simulink model "STATE_PROJECT"  (R2022b)
settings: Solver=FixedStepAuto  StartTime=0.0  StopTime=120.0  FixedStep=0.1  RelTol=1e-3
settings Model: Creator=alfon  LastModifiedBy=alfon

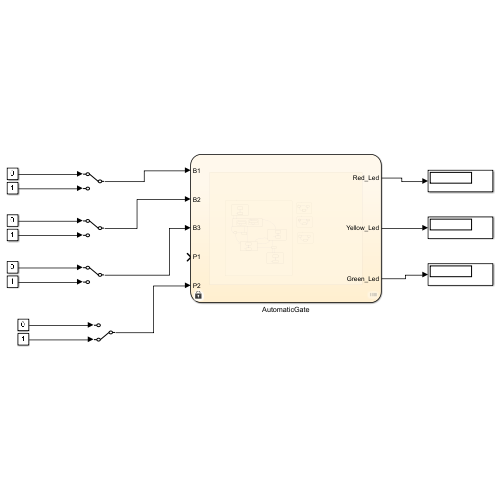
[thumbnail: Simulink's stored preview of the top-level diagram]
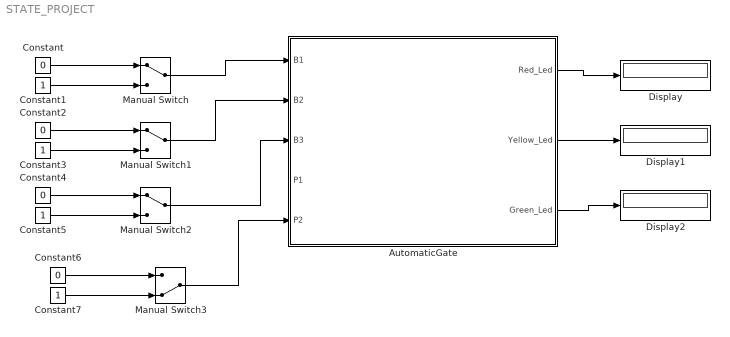
== system STATE_PROJECT ==
  AutomaticGate : Stateflow chart  TreatAsAtomicUnit=on
      settings: PortSchema="{\"entries\":[{\"content\":{\"sides\":[{\"content\":{\"connectorIds\":[\"In1\",\"In2\",\"In3\",\"In4\",\"In5\"]},\"type\":\"ConnectorPlacement.EquallySpacedRectSide\",\"uuid\":\"b9ac80a2-bb7a-47d7-8c7f-6386963f3ff2\"},{\"content\":{\"connectorIds\":[\"Out1\",\"Out3\",\"Out2\"],\"side\":\"RIGHT\"},\"type\":\"ConnectorPlacement.EquallySpacedRectSide\",\"uuid\":\"565990b0-d594-46a7-8ea3-0c7443a62f81\"},{\"content\":{\"connectorIds\":[],\"side\":\"TOP\"},\"type\":\"ConnectorPlacement.EquallySpacedRectSide\",\"uuid\":\"d7a99aca-bf8f-44a8-855e-79befe08fc9b\"}]},\"type\":\"ConnectorPlacement.EquallySpacedConnector\",\"uuid\":\"af0d90d0-169d-45ca-9585-d3b64258f7d0\"}],\"packageUris\":[\"http://schema.mathworks.com/mf0/Connector/R2020b\"],\"version\":\"1.0\"}"
  Constant{,2,4,6} (4 alike) : Constant  Value=0
  Constant{1,3,5,7} (4 alike) : Constant
  Display : Display
  Display1 : Display
  Display2 : Display
  Manual Switch : ManualSwitch
  Manual Switch1 : ManualSwitch
  Manual Switch2 : ManualSwitch
  Manual Switch3 : ManualSwitch  CurrentSetting=0
  wires:
  Constant/1 -> Manual Switch/1
  Constant1/1 -> Manual Switch/2
  Constant2/1 -> Manual Switch1/1
  Constant3/1 -> Manual Switch1/2
  Constant4/1 -> Manual Switch2/1
  Constant5/1 -> Manual Switch2/2
  Manual Switch/1 -> AutomaticGate/1(B1)
  Manual Switch1/1 -> AutomaticGate/2(B2)
  AutomaticGate/1(Red_Led) -> Display/1
  AutomaticGate/3(Yellow_Led) -> Display1/1
  AutomaticGate/2(Green_Led) -> Display2/1
  Constant7/1 -> Manual Switch3/2
  Constant6/1 -> Manual Switch3/1
  Manual Switch3/1 -> AutomaticGate/5(P2)
  Manual Switch2/1 -> AutomaticGate/3(B3)

== stateflow chart STATE_PROJECT/AutomaticGate ==
  state AUTOMATIC_GATE_LOGIC
    state AUTOMATIC_GATE [parallel]
      settings: executionOrder=4
      state EMERGENCY_P1_CLOSED
        state GREEN_OFF
          en:
          Green_Led = LED_OFF;
          Yellow_Led = LED_OFF;
          Red_Led = LED_OFF;
        state GREEN_ON
          en:
          Green_Led = LED_ON;
          Yellow_Led = LED_OFF;
          Red_Led = LED_OFF;
        AUTOMATIC_GATE_LOGIC.AUTOMATIC_GATE.EMERGENCY_P1_CLOSED.GREEN_ON -> AUTOMATIC_GATE_LOGIC.AUTOMATIC_GATE.EMERGENCY_P1_CLOSED.GREEN_OFF : [after(GREEN_DUR,sec)]
        AUTOMATIC_GATE_LOGIC.AUTOMATIC_GATE.EMERGENCY_P1_CLOSED.GREEN_OFF -> AUTOMATIC_GATE_LOGIC.AUTOMATIC_GATE.EMERGENCY_P1_CLOSED.GREEN_ON : [after(GREEN_DUR,sec)]
        (default) -> AUTOMATIC_GATE_LOGIC.AUTOMATIC_GATE.EMERGENCY_P1_CLOSED.GREEN_ON
      state CLOSED
        en:
        Green_Led = LED_OFF;
        Yellow_Led = LED_OFF;
        Red_Led = LED_OFF;
        state WORK_DUR_SETTING [parallel]
          settings: executionOrder=2
          state WORK_DUR_SETTING_INTERNAL
          (default) -> WORK_DUR_SETTING_INTERNAL
          WORK_DUR_SETTING_INTERNAL -> WORK_DUR_SETTING_INTERNAL : B3_pressed{WORK_DUR = mod((WORK_DUR),120) +10;}
        state OPEN_DUR_SETTING [parallel]
          settings: executionOrder=1
          state OPEN_DUR_SETTING_INTERNAL
          OPEN_DUR_SETTING_INTERNAL -> OPEN_DUR_SETTING_INTERNAL : B2_pressed{OPEN_DUR = mod((OPEN_DUR),120) + 10;}
        (default) -> WORK_DUR_SETTING [order 2]
        (default) -> OPEN_DUR_SETTING [order 1]
      state OPENING
        state YELLOW_OFF
          en:
          Green_Led = LED_OFF;
          Yellow_Led = LED_OFF;
          Red_Led = LED_OFF;
        state YELLOW_ON
          en:
          Green_Led = LED_OFF;
          Yellow_Led = LED_ON;
          Red_Led = LED_OFF;
        AUTOMATIC_GATE_LOGIC.AUTOMATIC_GATE.OPENING.YELLOW_ON -> AUTOMATIC_GATE_LOGIC.AUTOMATIC_GATE.OPENING.YELLOW_OFF : [after(YELLOW_DUR,sec)]
        AUTOMATIC_GATE_LOGIC.AUTOMATIC_GATE.OPENING.YELLOW_OFF -> AUTOMATIC_GATE_LOGIC.AUTOMATIC_GATE.OPENING.YELLOW_ON : [after(YELLOW_DUR,sec)]
        (default) -> AUTOMATIC_GATE_LOGIC.AUTOMATIC_GATE.OPENING.YELLOW_ON
      state EMERGENCY
        en:
        Green_Led = LED_OFF;
        Yellow_Led = LED_OFF;
        Red_Led = LED_OFF;
      state EMERGENCY_LED
        en:
        Green_Led = LED_OFF;
        Yellow_Led = LED_OFF;
        Red_Led = LED_ON;
      state CLOSING
        state YELLOW_OFF
          en:
          Green_Led = LED_OFF;
          Yellow_Led = LED_OFF;
          Red_Led = LED_OFF;
        state YELLOW_ON
          en:
          Green_Led = LED_OFF;
          Yellow_Led = LED_ON;
          Red_Led = LED_OFF;
        AUTOMATIC_GATE_LOGIC.AUTOMATIC_GATE.CLOSING.YELLOW_ON -> AUTOMATIC_GATE_LOGIC.AUTOMATIC_GATE.CLOSING.YELLOW_OFF : [after(YELLOW_DUR,sec)]
        AUTOMATIC_GATE_LOGIC.AUTOMATIC_GATE.CLOSING.YELLOW_OFF -> AUTOMATIC_GATE_LOGIC.AUTOMATIC_GATE.CLOSING.YELLOW_ON : [after(YELLOW_DUR,sec)]
        (default) -> AUTOMATIC_GATE_LOGIC.AUTOMATIC_GATE.CLOSING.YELLOW_ON
      state OPEN
        en:
        Green_Led = LED_ON;
        Yellow_Led = LED_ON;
        Red_Led = LED_ON;
      state EMERGENCY_P1_OPEN
        state GREEN_OFF
          en:
          Green_Led = LED_OFF;
          Yellow_Led = LED_OFF;
          Red_Led = LED_OFF;
        state GREEN_ON
          en:
          Green_Led = LED_ON;
          Yellow_Led = LED_OFF;
          Red_Led = LED_OFF;
        AUTOMATIC_GATE_LOGIC.AUTOMATIC_GATE.EMERGENCY_P1_OPEN.GREEN_ON -> AUTOMATIC_GATE_LOGIC.AUTOMATIC_GATE.EMERGENCY_P1_OPEN.GREEN_OFF : [after(GREEN_DUR,sec)]
        AUTOMATIC_GATE_LOGIC.AUTOMATIC_GATE.EMERGENCY_P1_OPEN.GREEN_OFF -> AUTOMATIC_GATE_LOGIC.AUTOMATIC_GATE.EMERGENCY_P1_OPEN.GREEN_ON : [after(GREEN_DUR,sec)]
        (default) -> AUTOMATIC_GATE_LOGIC.AUTOMATIC_GATE.EMERGENCY_P1_OPEN.GREEN_ON
      CLOSED -> EMERGENCY_P1_CLOSED [order 1] : [B1_pressed && P1 == P_ON]
      EMERGENCY_P1_CLOSED -> CLOSED : [P1 == P_OFF || after(EMER_P1_DUR,sec)]
      CLOSED -> OPENING [order 2] : B1_pressed
      EMERGENCY -> CLOSED [order 2] : [P2 == P_ON]
      EMERGENCY_LED -> CLOSED : [P2 == P_ON]
      CLOSING -> CLOSED [order 1] : [P2 == P_ON]
      EMERGENCY -> EMERGENCY_LED [order 1] : [after(EMER_DUR,sec)]
      CLOSING -> EMERGENCY [order 3] : [after(WORK_DUR,sec)]
      OPENING -> CLOSING [order 1] : [B1_pressed && P1 == P_OFF]
      CLOSING -> OPENING [order 2] : [B1_pressed || P1 == P_ON]
      OPENING -> OPEN [order 2] : [after(WORK_DUR,sec)]
      (default) -> CLOSING
      OPEN -> CLOSING [order 1] : [after(OPEN_DUR,sec) || B1_pressed]
      EMERGENCY_P1_OPEN -> OPEN : [P1 == P_OFF || after(EMER_P1_DUR,sec)]
      OPEN -> EMERGENCY_P1_OPEN [order 2] : [B1_pressed && P1 == P_ON]
    state B1 [parallel]
      settings: executionOrder=1
      state RELEASED
      state PRESSED
      state LONGPRESSED
        send(B1_pressed)
      (default) -> AUTOMATIC_GATE_LOGIC.B1.RELEASED
      AUTOMATIC_GATE_LOGIC.B1.RELEASED -> AUTOMATIC_GATE_LOGIC.B1.PRESSED : [B1==BUTTON_ON]
      AUTOMATIC_GATE_LOGIC.B1.LONGPRESSED -> AUTOMATIC_GATE_LOGIC.B1.RELEASED : [B1 == BUTTON_OFF]
      AUTOMATIC_GATE_LOGIC.B1.PRESSED -> AUTOMATIC_GATE_LOGIC.B1.LONGPRESSED : [B1 == BUTTON_OFF]
    state B3 [parallel]
      settings: executionOrder=2
      state RELEASED
      state PRESSED
      state LONGPRESSED
        send(B3_pressed)
      (default) -> AUTOMATIC_GATE_LOGIC.B3.RELEASED
      AUTOMATIC_GATE_LOGIC.B3.RELEASED -> AUTOMATIC_GATE_LOGIC.B3.PRESSED : [B3==BUTTON_ON]
      AUTOMATIC_GATE_LOGIC.B3.LONGPRESSED -> AUTOMATIC_GATE_LOGIC.B3.RELEASED : [B3 == BUTTON_OFF]
      AUTOMATIC_GATE_LOGIC.B3.PRESSED -> AUTOMATIC_GATE_LOGIC.B3.LONGPRESSED : [B3== BUTTON_OFF]
    state B2 [parallel]
      settings: executionOrder=3
      state RELEASED
      state PRESSED
      state LONGPRESSED
        send(B2_pressed)
      (default) -> AUTOMATIC_GATE_LOGIC.B2.RELEASED
      AUTOMATIC_GATE_LOGIC.B2.RELEASED -> AUTOMATIC_GATE_LOGIC.B2.PRESSED : [B2==BUTTON_ON]
      AUTOMATIC_GATE_LOGIC.B2.LONGPRESSED -> AUTOMATIC_GATE_LOGIC.B2.RELEASED : [B2 == BUTTON_OFF]
      AUTOMATIC_GATE_LOGIC.B2.PRESSED -> AUTOMATIC_GATE_LOGIC.B2.LONGPRESSED : [B2 == BUTTON_OFF]
    (default) -> AUTOMATIC_GATE [order 1]
    (default) -> B1 [order 2]
    (default) -> B3 [order 4]
    (default) -> B2 [order 3]
  data: B1 input; B2 input; B3 input; Red_Led output; Green_Led output; Yellow_Led output; P1 input; P2 input; BUTTON_OFF constant double =0; WORK_DUR local =10; P_ON constant double =1; P_OFF constant double =0; OPEN_DUR local =10; LED_ON constant double =1; LED_OFF constant double =0; BUTTON_ON constant double =1; EMER_DUR constant double =10; YELLOW_DUR constant double =1; GREEN_DUR constant double =0.5; EMER_P1_DUR constant double =30
  events: B1_pressed local RISING_EDGE_EVENT; B2_pressed local FUNCTION_CALL_EVENT; B3_pressed local FUNCTION_CALL_EVENT
